simulink model "TCGreen"  (R2024b)
settings: Solver=ode45  StartTime=0.0  StopTime=1  RelTol=1e-3
undefined symbols (not defined in the file or in its folder): Cf, F, Kic, Kiv, Kpc, Kpv, Lc, Lf, Lline, mp, nq, rc, rf, Rline, Rload, Ts, Vdc, Vn, wc, wn
libraries: spsFourierLib x18, spsabctodq0Lib x14, spsThreePhaseSeriesRLCBranchLib x13, spsThreePhaseVIMeasurementLib x11, spsGroundLib x5, simulink x3, spsDCVoltageSourceLib x3, spsUniversalBridgeLib x3, spsdq0toabcLib x3, sps_lib x1
settings Model: Creator=RDP  LastModifiedBy=DAS'BEAST
settings DataIOCC: ReturnWorkspaceOutputs=off
settings RTWCC: GPUComputeCapability=3.5

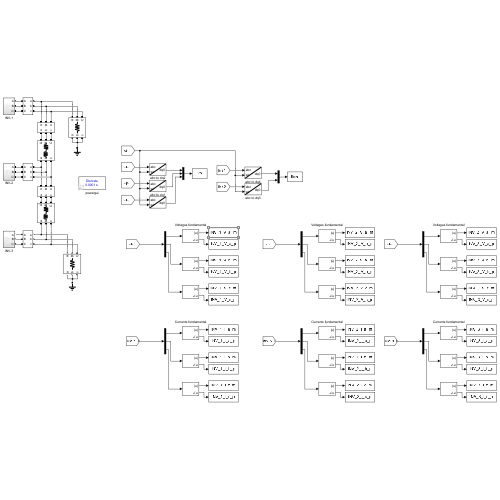
[thumbnail: Simulink's stored preview of the top-level diagram]
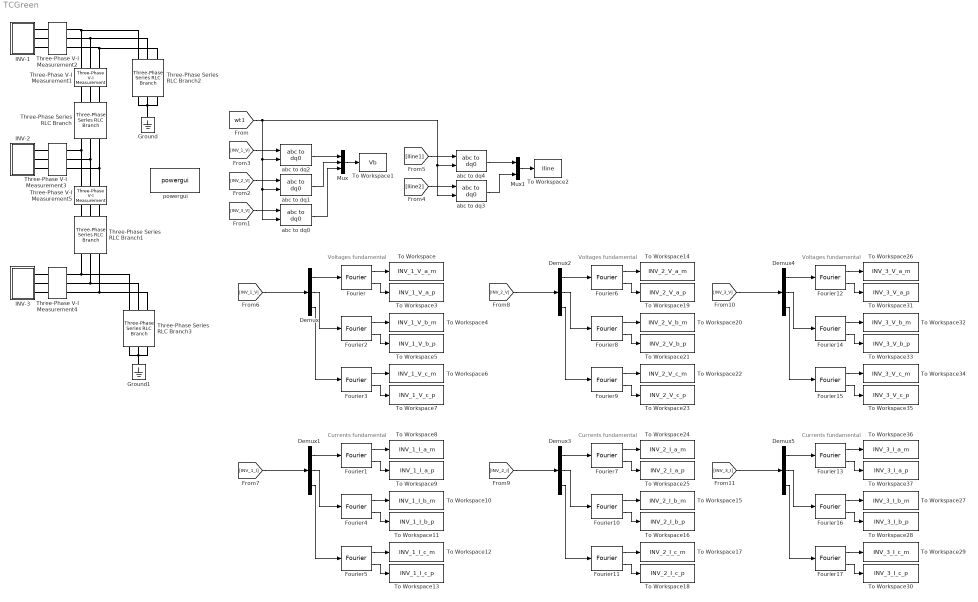
== system TCGreen ==
  note: Voltages fundamental
  note: Currents fundamental
  note: Currents fundamental
  note: Voltages fundamental
  note: Currents fundamental
  note: Voltages fundamental
  Demux{,1..5} (6 alike) : Demux  Outputs=3
  Fourier{,1..17} (18 alike) : spsFourierLib/Fourier  Freq=50  n=1  InInit=[0, 0]  Ts=0
  Ground : spsGroundLib/Ground  LConnTagsString=a
  Ground1 : spsGroundLib/Ground  LConnTagsString=a
  INV-1 : Subsystem
  INV-2 : Subsystem
  INV-3 : Subsystem
  Mux : Mux  Inputs=3
  Mux1 : Mux  Inputs=2
  Three-Phase Series RLC Branch : spsThreePhaseSeriesRLCBranchLib/Three-Phase Series RLC Branch  LConnTagsString=A|B|C  RConnTagsString=A|B|C  BranchType=RL  Resistance=Rline(1)  Inductance=Lline(1)  Capacitance=1e-6  Measurements=None
  Three-Phase Series RLC Branch1 : spsThreePhaseSeriesRLCBranchLib/Three-Phase Series RLC Branch  LConnTagsString=A|B|C  RConnTagsString=A|B|C  BranchType=RL  Resistance=Rline(2)  Inductance=Lline(2)  Capacitance=1e-6  Measurements=None
  Three-Phase Series RLC Branch2 : spsThreePhaseSeriesRLCBranchLib/Three-Phase Series RLC Branch  LConnTagsString=A|B|C  RConnTagsString=A|B|C  BranchType=R  Resistance=Rload(1)  Inductance=Lline(1)  Capacitance=1e-6  Measurements=None
  Three-Phase Series RLC Branch3 : spsThreePhaseSeriesRLCBranchLib/Three-Phase Series RLC Branch  LConnTagsString=A|B|C  RConnTagsString=A|B|C  BranchType=R  Resistance=Rload(2)  Inductance=Lline(1)  Capacitance=1e-6  Measurements=None
  Three-Phase V-I Measurement1 : spsThreePhaseVIMeasurementLib/Three-Phase V-I Measurement  VoltageMeasurement=no  SetLabelV=on  LabelV=Vb1  Vpu=off  VpuLL=off  CurrentMeasurement=yes  SetLabelI=on  LabelI=Iline1  Ipu=off  Pbase=100e6  Vbase=500e3  OutputType=Complex  PhasorSimulation=off  PSBequivalent=0
  Three-Phase V-I Measurement2 : spsThreePhaseVIMeasurementLib/Three-Phase V-I Measurement  VoltageMeasurement=phase-to-ground  SetLabelV=on  LabelV=INV_1_V  Vpu=off  VpuLL=off  CurrentMeasurement=yes  SetLabelI=on  LabelI=INV_1_I  Ipu=off  Pbase=100e6  Vbase=500e3  OutputType=Complex  PhasorSimulation=off  PSBequivalent=0
  Three-Phase V-I Measurement3 : spsThreePhaseVIMeasurementLib/Three-Phase V-I Measurement  VoltageMeasurement=phase-to-ground  SetLabelV=on  LabelV=INV_2_V  Vpu=off  VpuLL=off  CurrentMeasurement=yes  SetLabelI=on  LabelI=INV_2_I  Ipu=off  Pbase=100e6  Vbase=500e3  OutputType=Complex  PhasorSimulation=off  PSBequivalent=0
  Three-Phase V-I Measurement4 : spsThreePhaseVIMeasurementLib/Three-Phase V-I Measurement  VoltageMeasurement=phase-to-ground  SetLabelV=on  LabelV=INV_3_V  Vpu=off  VpuLL=off  CurrentMeasurement=yes  SetLabelI=on  LabelI=INV_3_I  Ipu=off  Pbase=100e6  Vbase=500e3  OutputType=Complex  PhasorSimulation=off  PSBequivalent=0
  Three-Phase V-I Measurement5 : spsThreePhaseVIMeasurementLib/Three-Phase V-I Measurement  VoltageMeasurement=no  SetLabelV=on  LabelV=Vb1  Vpu=off  VpuLL=off  CurrentMeasurement=yes  SetLabelI=on  LabelI=Iline2  Ipu=off  Pbase=100e6  Vbase=500e3  OutputType=Complex  PhasorSimulation=off  PSBequivalent=0
  To Workspace : ToWorkspace  VariableName=INV_1_V_a_m  SaveFormat=Timeseries  SampleTime=-1
  To Workspace1 : ToWorkspace  VariableName=Vb  SampleTime=-1
      settings: MaxDataPoints=1  Save2DSignal=2-D array (concatenate along first dimension)
  To Workspace10 : ToWorkspace  VariableName=INV_1_I_b_m  SaveFormat=Timeseries  SampleTime=-1
  To Workspace11 : ToWorkspace  VariableName=INV_1_I_b_p  SaveFormat=Timeseries  SampleTime=-1
  To Workspace12 : ToWorkspace  VariableName=INV_1_I_c_m  SaveFormat=Timeseries  SampleTime=-1
  To Workspace13 : ToWorkspace  VariableName=INV_1_I_c_p  SaveFormat=Timeseries  SampleTime=-1
  To Workspace14 : ToWorkspace  VariableName=INV_2_V_a_m  SaveFormat=Timeseries  SampleTime=-1
  To Workspace15 : ToWorkspace  VariableName=INV_2_I_b_m  SaveFormat=Timeseries  SampleTime=-1
  To Workspace16 : ToWorkspace  VariableName=INV_2_I_b_p  SaveFormat=Timeseries  SampleTime=-1
  To Workspace17 : ToWorkspace  VariableName=INV_2_I_c_m  SaveFormat=Timeseries  SampleTime=-1
  To Workspace18 : ToWorkspace  VariableName=INV_2_I_c_p  SaveFormat=Timeseries  SampleTime=-1
  To Workspace19 : ToWorkspace  VariableName=INV_2_V_a_p  SaveFormat=Timeseries  SampleTime=-1
  To Workspace2 : ToWorkspace  VariableName=Iline  SampleTime=-1
      settings: MaxDataPoints=1  Save2DSignal=2-D array (concatenate along first dimension)
  To Workspace20 : ToWorkspace  VariableName=INV_2_V_b_m  SaveFormat=Timeseries  SampleTime=-1
  To Workspace21 : ToWorkspace  VariableName=INV_2_V_b_p  SaveFormat=Timeseries  SampleTime=-1
  To Workspace22 : ToWorkspace  VariableName=INV_2_V_c_m  SaveFormat=Timeseries  SampleTime=-1
  To Workspace23 : ToWorkspace  VariableName=INV_2_V_c_p  SaveFormat=Timeseries  SampleTime=-1
  To Workspace24 : ToWorkspace  VariableName=INV_2_I_a_m  SaveFormat=Timeseries  SampleTime=-1
  To Workspace25 : ToWorkspace  VariableName=INV_2_I_a_p  SaveFormat=Timeseries  SampleTime=-1
  To Workspace26 : ToWorkspace  VariableName=INV_3_V_a_m  SaveFormat=Timeseries  SampleTime=-1
  To Workspace27 : ToWorkspace  VariableName=INV_3_I_b_m  SaveFormat=Timeseries  SampleTime=-1
  To Workspace28 : ToWorkspace  VariableName=INV_3_I_b_p  SaveFormat=Timeseries  SampleTime=-1
  To Workspace29 : ToWorkspace  VariableName=INV_3_I_c_m  SaveFormat=Timeseries  SampleTime=-1
  To Workspace3 : ToWorkspace  VariableName=INV_1_V_a_p  SaveFormat=Timeseries  SampleTime=-1
  To Workspace30 : ToWorkspace  VariableName=INV_3_I_c_p  SaveFormat=Timeseries  SampleTime=-1
  To Workspace31 : ToWorkspace  VariableName=INV_3_V_a_p  SaveFormat=Timeseries  SampleTime=-1
  To Workspace32 : ToWorkspace  VariableName=INV_3_V_b_m  SaveFormat=Timeseries  SampleTime=-1
  To Workspace33 : ToWorkspace  VariableName=INV_3_V_b_p  SaveFormat=Timeseries  SampleTime=-1
  To Workspace34 : ToWorkspace  VariableName=INV_3_V_c_m  SaveFormat=Timeseries  SampleTime=-1
  To Workspace35 : ToWorkspace  VariableName=INV_3_V_c_p  SaveFormat=Timeseries  SampleTime=-1
  To Workspace36 : ToWorkspace  VariableName=INV_3_I_a_m  SaveFormat=Timeseries  SampleTime=-1
  To Workspace37 : ToWorkspace  VariableName=INV_3_I_a_p  SaveFormat=Timeseries  SampleTime=-1
  To Workspace4 : ToWorkspace  VariableName=INV_1_V_b_m  SaveFormat=Timeseries  SampleTime=-1
  To Workspace5 : ToWorkspace  VariableName=INV_1_V_b_p  SaveFormat=Timeseries  SampleTime=-1
  To Workspace6 : ToWorkspace  VariableName=INV_1_V_c_m  SaveFormat=Timeseries  SampleTime=-1
  To Workspace7 : ToWorkspace  VariableName=INV_1_V_c_p  SaveFormat=Timeseries  SampleTime=-1
  To Workspace8 : ToWorkspace  VariableName=INV_1_I_a_m  SaveFormat=Timeseries  SampleTime=-1
  To Workspace9 : ToWorkspace  VariableName=INV_1_I_a_p  SaveFormat=Timeseries  SampleTime=-1
  abc to dq{0..4} (5 alike) : spsabctodq0Lib/abc to dq0  Alignment=90 degrees behind phase A axis
  powergui : sps_lib/powergui  Priority=1  SimulationMode=Discrete  SampleTime=Ts  frequency=60  Iterations=50  frequencyindice=0  Pbase=100e6  ErrMax=1e-4  UnitsV=kV  UnitsW=MW  buscounter=0  FunctionMessages=off  echomessages=off  EnableUseOfTLC=off  CurrentSourceSwitches=off  DisableSnubberDevices=off  DisableRonSwitches=off  DisableVfSwitches=off  DisplayEquations=off  AutomaticDiscreteSolvers=off  SolverType=Tustin/Backward Euler (TBE)  Interpol=off  ExternalGateDelay=off  methode=off  Ts=100  x0status=blocks  SPID=on  SwTol=0  HookPort=off  NonlinearTolerance=1e-4  nMaxIteration=100  ContinueOnMaxIteration=off  RestoreLinks=warning  ResistiveCurrentMeasurement=off  Frange=[0:2:500]  Ylog=off  Xlog=on  ShowGrid=off  save=off  variable=ZData  structure=0  ZoomFFT=off  StartTime=0.0  cycles=1  DisplayStyle=1  fundamental=60  FreqAxis=off  MaxFrequency=1000  frequencyindicesteady=1  RmsSteady=1  display=off
  wires:
  [INV_3_V] -> abc to dq0/1
  [INV_2_V] -> abc to dq1/1
  [INV_1_V] -> abc to dq2/1
  abc to dq2/1 -> Mux/1
  abc to dq1/1 -> Mux/2
  abc to dq0/1 -> Mux/3
  Mux/1 -> To Workspace1/1
  Mux1/1 -> To Workspace2/1
  abc to dq3/1 -> Mux1/2
  abc to dq4/1 -> Mux1/1
  [Iline1] -> abc to dq4/1
  [Iline2] -> abc to dq3/1
  [wt1] -> abc to dq3/2, abc to dq4/2, abc to dq2/2, abc to dq0/2, abc to dq1/2
  [INV_1_V] -> Demux/1
  Demux/2 -> Fourier2/1
  Demux/3 -> Fourier3/1
  Demux/1 -> Fourier/1
  Fourier/1 -> To Workspace/1
  Fourier2/1 -> To Workspace4/1
  Fourier3/1 -> To Workspace6/1
  Fourier3/2 -> To Workspace7/1
  Fourier2/2 -> To Workspace5/1
  Fourier/2 -> To Workspace3/1
  Demux1/1 -> Fourier1/1
  Demux1/2 -> Fourier4/1
  Fourier4/1 -> To Workspace10/1
  Fourier5/2 -> To Workspace13/1
  Fourier1/1 -> To Workspace8/1
  Fourier5/1 -> To Workspace12/1
  Demux1/3 -> Fourier5/1
  Fourier4/2 -> To Workspace11/1
  [INV_1_I] -> Demux1/1
  Fourier1/2 -> To Workspace9/1
  Demux2/1 -> Fourier6/1
  Demux2/2 -> Fourier8/1
  Fourier8/2 -> To Workspace21/1
  Fourier8/1 -> To Workspace20/1
  Demux3/3 -> Fourier11/1
  Fourier10/2 -> To Workspace16/1
  Fourier7/2 -> To Workspace25/1
  Fourier11/1 -> To Workspace17/1
  [INV_2_I] -> Demux3/1
  Demux3/2 -> Fourier10/1
  Fourier11/2 -> To Workspace18/1
  Fourier9/2 -> To Workspace23/1
  Fourier6/1 -> To Workspace14/1
  Demux3/1 -> Fourier7/1
  Fourier9/1 -> To Workspace22/1
  Demux2/3 -> Fourier9/1
  Fourier10/1 -> To Workspace15/1
  Fourier6/2 -> To Workspace19/1
  [INV_2_V] -> Demux2/1
  Fourier7/1 -> To Workspace24/1
  Demux4/1 -> Fourier12/1
  Demux4/2 -> Fourier14/1
  Fourier14/2 -> To Workspace33/1
  Fourier14/1 -> To Workspace32/1
  Demux5/3 -> Fourier17/1
  Fourier16/2 -> To Workspace28/1
  Fourier13/2 -> To Workspace37/1
  Fourier17/1 -> To Workspace29/1
  [INV_3_I] -> Demux5/1
  Demux5/2 -> Fourier16/1
  Fourier17/2 -> To Workspace30/1
  Fourier15/2 -> To Workspace35/1
  Fourier12/1 -> To Workspace26/1
  Demux5/1 -> Fourier13/1
  Fourier15/1 -> To Workspace34/1
  Demux4/3 -> Fourier15/1
  Fourier16/1 -> To Workspace27/1
  Fourier12/2 -> To Workspace31/1
  [INV_3_V] -> Demux4/1
  Fourier13/1 -> To Workspace36/1
  connections:
  Three-Phase Series RLC Branch2/LConn1 -- Three-Phase V-I Measurement2/RConn1 -- Three-Phase V-I Measurement1/LConn1
  Three-Phase V-I Measurement2/RConn2 -- Three-Phase V-I Measurement1/LConn2 -- Three-Phase Series RLC Branch2/LConn2
  Three-Phase Series RLC Branch2/LConn3 -- Three-Phase V-I Measurement1/LConn3 -- Three-Phase V-I Measurement2/RConn3
  Three-Phase V-I Measurement3/RConn1 -- Three-Phase V-I Measurement5/LConn1 -- Three-Phase Series RLC Branch/RConn1
  Three-Phase V-I Measurement3/RConn2 -- Three-Phase V-I Measurement5/LConn2 -- Three-Phase Series RLC Branch/RConn2
  Three-Phase V-I Measurement3/RConn3 -- Three-Phase V-I Measurement5/LConn3 -- Three-Phase Series RLC Branch/RConn3
  Three-Phase Series RLC Branch2/RConn1 -- Ground/LConn1 -- Three-Phase Series RLC Branch2/RConn2 -- Three-Phase Series RLC Branch2/RConn3
  Three-Phase Series RLC Branch1/RConn1 -- Three-Phase Series RLC Branch3/LConn1 -- Three-Phase V-I Measurement4/RConn1
  Three-Phase Series RLC Branch1/RConn2 -- Three-Phase V-I Measurement4/RConn2 -- Three-Phase Series RLC Branch3/LConn2
  Three-Phase Series RLC Branch1/RConn3 -- Three-Phase Series RLC Branch3/LConn3 -- Three-Phase V-I Measurement4/RConn3
  Three-Phase Series RLC Branch3/RConn1 -- Ground1/LConn1 -- Three-Phase Series RLC Branch3/RConn2 -- Three-Phase Series RLC Branch3/RConn3
  INV-1/RConn1 -- Three-Phase V-I Measurement2/LConn1
  INV-1/RConn2 -- Three-Phase V-I Measurement2/LConn2
  INV-1/RConn3 -- Three-Phase V-I Measurement2/LConn3
  Three-Phase V-I Measurement3/LConn1 -- INV-2/RConn1
  Three-Phase V-I Measurement3/LConn2 -- INV-2/RConn2
  Three-Phase V-I Measurement3/LConn3 -- INV-2/RConn3
  Three-Phase V-I Measurement4/LConn1 -- INV-3/RConn1
  Three-Phase V-I Measurement4/LConn2 -- INV-3/RConn2
  Three-Phase V-I Measurement4/LConn3 -- INV-3/RConn3
  Three-Phase V-I Measurement1/RConn1 -- Three-Phase Series RLC Branch/LConn1
  Three-Phase Series RLC Branch/LConn2 -- Three-Phase V-I Measurement1/RConn2
  Three-Phase V-I Measurement1/RConn3 -- Three-Phase Series RLC Branch/LConn3
  Three-Phase V-I Measurement5/RConn1 -- Three-Phase Series RLC Branch1/LConn1
  Three-Phase V-I Measurement5/RConn2 -- Three-Phase Series RLC Branch1/LConn2
  Three-Phase V-I Measurement5/RConn3 -- Three-Phase Series RLC Branch1/LConn3

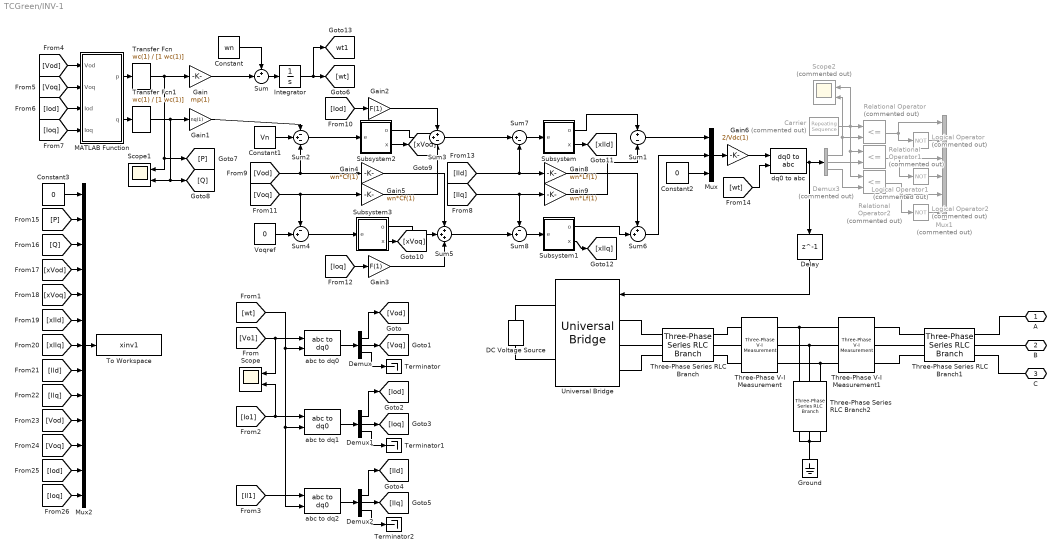
== system TCGreen/INV-1 ==
  Carrier : simulink/Sources/Repeating Sequence  Commented=on  rep_seq_t=[0 0.5 1]/10000  rep_seq_y=[-1 1 -1]
  Constant : Constant  Value=wn
  Constant1 : Constant  Value=Vn
  Constant2 : Constant  Value=0
  Constant3 : Constant  Value=0
  DC Voltage Source : spsDCVoltageSourceLib/DC Voltage Source  Amplitude=Vdc(1)  Measurements=None
  Delay : Delay  DelayLength=1
  Demux : Demux  Outputs=3
  Demux1 : Demux  Outputs=3
  Demux2 : Demux  Outputs=3
  Demux3 : Demux  Commented=on  Outputs=3
  Gain : Gain  Gain=mp(1)
  Gain1 : Gain  Gain=nq(1)
  Gain2 : Gain  Gain=F(1)
  Gain3 : Gain  Gain=F(1)
  Gain4 : Gain  Gain=wn*Cf(1)
  Gain5 : Gain  Gain=wn*Cf(1)
  Gain6 : Gain  Gain=2/Vdc(1)
  Gain8 : Gain  Gain=wn*Lf(1)
  Gain9 : Gain  Gain=wn*Lf(1)
  Ground : spsGroundLib/Ground  LConnTagsString=a
  Integrator : Integrator  WrappedStateUpperValue=2*pi  WrappedStateLowerValue=0
  Logical Operator : Logic  Commented=on  Operator=NOT  IconShape=distinctive  AllPortsSameDT=off  OutDataTypeStr=boolean
  Logical Operator1 : Logic  Commented=on  Operator=NOT  IconShape=distinctive  AllPortsSameDT=off  OutDataTypeStr=boolean
  Logical Operator2 : Logic  Commented=on  Operator=NOT  IconShape=distinctive  AllPortsSameDT=off  OutDataTypeStr=boolean
  MATLAB Function : MATLAB Function  TreatAsAtomicUnit=on
  Mux : Mux  Inputs=3
  Mux1 : Mux  Commented=on  Inputs=6
  Mux2 : Mux  Inputs=13
  Relational Operator : RelationalOperator  Commented=on  Operator=<=  OutDataTypeStr=boolean  RndMeth=Simplest  InputSameDT=off
  Relational Operator1 : RelationalOperator  Commented=on  Operator=<=  OutDataTypeStr=boolean  RndMeth=Simplest  InputSameDT=off
  Relational Operator2 : RelationalOperator  Commented=on  Operator=<=  OutDataTypeStr=boolean  RndMeth=Simplest  InputSameDT=off
  Scope : Scope  NumInputPorts=2
  Scope1 : Scope  NumInputPorts=2
  Scope2 : Scope  Commented=on  NumInputPorts=2
  Subsystem : Subsystem
  Subsystem1 : Subsystem
  Subsystem2 : Subsystem
  Subsystem3 : Subsystem
  Sum : Sum  Inputs=+-|
  Sum1 : Sum  Inputs=+-
  Sum2 : Sum  Inputs=-+-
  Sum3 : Sum  Inputs=++-
  Sum4 : Sum  Inputs=-+|
  Sum5 : Sum  Inputs=+++
  Sum6 : Sum  Inputs=++|
  Sum7 : Sum  Inputs=|+-
  Sum8 : Sum  Inputs=-+|
  Terminator : Terminator
  Terminator1 : Terminator
  Terminator2 : Terminator
  Three-Phase Series RLC Branch : spsThreePhaseSeriesRLCBranchLib/Three-Phase Series RLC Branch  LConnTagsString=A|B|C  RConnTagsString=A|B|C  BranchType=RL  Resistance=rf(1)  Inductance=Lf(1)  Capacitance=1e-6  Measurements=None
  Three-Phase Series RLC Branch1 : spsThreePhaseSeriesRLCBranchLib/Three-Phase Series RLC Branch  LConnTagsString=A|B|C  RConnTagsString=A|B|C  BranchType=RL  Resistance=rc(1)  Inductance=Lc(1)  Capacitance=1e-6  Measurements=None
  Three-Phase Series RLC Branch2 : spsThreePhaseSeriesRLCBranchLib/Three-Phase Series RLC Branch  LConnTagsString=A|B|C  RConnTagsString=A|B|C  BranchType=C  Resistance=rf(1)  Inductance=Lf(1)  Capacitance=Cf(1)  Measurements=None
  Three-Phase V-I Measurement : spsThreePhaseVIMeasurementLib/Three-Phase V-I Measurement  VoltageMeasurement=no  SetLabelV=off  LabelV=Vabc  Vpu=off  VpuLL=off  CurrentMeasurement=yes  SetLabelI=on  LabelI=Il1  Ipu=off  Pbase=100e6  Vbase=500e3  OutputType=Complex  PhasorSimulation=off  PSBequivalent=0
  Three-Phase V-I Measurement1 : spsThreePhaseVIMeasurementLib/Three-Phase V-I Measurement  VoltageMeasurement=phase-to-ground  SetLabelV=on  LabelV=Vo1  Vpu=off  VpuLL=off  CurrentMeasurement=yes  SetLabelI=on  LabelI=Io1  Ipu=off  Pbase=100e6  Vbase=500e3  OutputType=Complex  PhasorSimulation=off  PSBequivalent=0
  To Workspace : ToWorkspace  VariableName=xinv1  SampleTime=-1
      settings: MaxDataPoints=1  Save2DSignal=2-D array (concatenate along first dimension)
  Transfer Fcn : TransferFcn  Numerator=wc(1)  Denominator=[1 wc(1)]
  Transfer Fcn1 : TransferFcn  Numerator=wc(1)  Denominator=[1 wc(1)]
  Universal Bridge : spsUniversalBridgeLib/Universal Bridge  Arms=3  SnubberResistance=1e5  SnubberCapacitance=inf  Device=Average-model based VSC  Ron=1e-3  Lon=0  ForwardVoltages="[  0  0  ]"  ForwardVoltage=0  GTOparameters=[ 10e-6 , 20e-6 ]  IGBTparameters=[ 1e-6 , 2e-6 ]  Measurements=None  Measurements_2=None  converterType=Rectifier
  Voqref : Constant  Value=0
  abc to dq0 : spsabctodq0Lib/abc to dq0  Alignment=90 degrees behind phase A axis
  abc to dq1 : spsabctodq0Lib/abc to dq0  Alignment=90 degrees behind phase A axis
  abc to dq2 : spsabctodq0Lib/abc to dq0  Alignment=90 degrees behind phase A axis
  dq0 to abc : spsdq0toabcLib/dq0 to abc  Alignment=90 degrees behind phase A axis
  A : PMIOPort  Side=Right
  B : PMIOPort  Port=2  Side=Right
  C : PMIOPort  Port=3  Side=Right
  tag scope: wt1=global
  wires:
  [Vo1] -> Scope/1, abc to dq0/1
  abc to dq0/1 -> Demux/1
  Demux/1 -> [Vod]
  Demux/2 -> [Voq]
  Demux/3 -> Terminator/1
  Demux1/3 -> Terminator1/1
  Demux1/2 -> [Ioq]
  Demux1/1 -> [Iod]
  abc to dq1/1 -> Demux1/1
  [Io1] -> Scope/2, abc to dq1/1
  [Il1] -> abc to dq2/1
  Demux2/1 -> [Ild]
  abc to dq2/1 -> Demux2/1
  Demux2/2 -> [Ilq]
  Demux2/3 -> Terminator2/1
  [wt] -> abc to dq0/2, abc to dq1/2, abc to dq2/2
  [Voq] -> MATLAB Function/2(Voq)
  [Vod] -> MATLAB Function/1(Vod)
  [Iod] -> MATLAB Function/3(Iod)
  [Ioq] -> MATLAB Function/4(Ioq)
  MATLAB Function/1(p) -> Transfer Fcn/1
  MATLAB Function/2(q) -> Transfer Fcn1/1
  Transfer Fcn/1 -> Scope1/1, [P], Gain/1
  Constant/1 -> Sum/1
  Transfer Fcn1/1 -> [Q], Scope1/2, Gain1/1
  Sum/1 -> Integrator/1
  Integrator/1 -> [wt], [wt1]
  [Vod] -> Sum2/3, Gain4/1
  Sum2/1 -> Subsystem2/1(e)
  Subsystem2/1(o) -> Sum3/2
  [Iod] -> Gain2/1
  Gain2/1 -> Sum3/1
  Voqref/1 -> Sum4/2
  [Voq] -> Gain5/1, Sum4/1
  Sum4/1 -> Subsystem3/1(e)
  Subsystem3/1(o) -> Sum5/2
  [Ioq] -> Gain3/1
  Gain3/1 -> Sum5/3
  Gain4/1 -> Sum5/1
  Gain5/1 -> Sum3/3
  Constant1/1 -> Sum2/2
  Gain8/1 -> Sum6/1
  Subsystem1/1(o) -> Sum6/2
  [Ilq] -> Sum8/1, Gain9/1
  [Ild] -> Sum7/2, Gain8/1
  Subsystem/1(o) -> Sum1/1
  Gain9/1 -> Sum1/2
  Sum3/1 -> Sum7/1
  Sum5/1 -> Sum8/2
  Sum7/1 -> Subsystem/1(e)
  Sum8/1 -> Subsystem1/1(e)
  Sum1/1 -> Mux/1
  Sum6/1 -> Mux/2
  Constant2/1 -> Mux/3
  Mux/1 -> Gain6/1
  Gain6/1 -> dq0 to abc/1
  [wt] -> dq0 to abc/2
  dq0 to abc/1 -> Demux3/1, Delay/1
  Demux3/1 -> Scope2/2, Relational Operator/2
  Demux3/2 -> Relational Operator1/2
  Demux3/3 -> Relational Operator2/2
  Carrier/1 -> Scope2/1, Relational Operator2/1, Relational Operator1/1, Relational Operator/1
  Relational Operator/1 -> Logical Operator/1, Mux1/1
  Relational Operator1/1 -> Logical Operator1/1, Mux1/3
  Relational Operator2/1 -> Logical Operator2/1, Mux1/5
  Logical Operator/1 -> Mux1/2
  Logical Operator1/1 -> Mux1/4
  Logical Operator2/1 -> Mux1/6
  Gain/1 -> Sum/2
  Gain1/1 -> Sum2/1
  Constant3/1 -> Mux2/1
  [P] -> Mux2/2
  [Q] -> Mux2/3
  [xVod] -> Mux2/4
  [xVoq] -> Mux2/5
  [xIld] -> Mux2/6
  [xIlq] -> Mux2/7
  [Ild] -> Mux2/8
  [Ilq] -> Mux2/9
  [Vod] -> Mux2/10
  [Voq] -> Mux2/11
  [Iod] -> Mux2/12
  [Ioq] -> Mux2/13
  Mux2/1 -> To Workspace/1
  Delay/1 -> Universal Bridge/1
  Subsystem/2(x) -> [xIld]
  Subsystem1/2(x) -> [xIlq]
  Subsystem2/2(x) -> [xVod]
  Subsystem3/2(x) -> [xVoq]
  connections:
  Three-Phase Series RLC Branch/LConn3 -- Universal Bridge/LConn3
  Three-Phase V-I Measurement/LConn3 -- Three-Phase Series RLC Branch/RConn3
  Three-Phase Series RLC Branch/RConn2 -- Three-Phase V-I Measurement/LConn2
  Three-Phase Series RLC Branch1/RConn3 -- C/RConn1
  Three-Phase Series RLC Branch/LConn2 -- Universal Bridge/LConn2
  Three-Phase V-I Measurement1/LConn2 -- Three-Phase V-I Measurement/RConn2 -- Three-Phase Series RLC Branch2/LConn2
  DC Voltage Source/RConn1 -- Universal Bridge/RConn1
  Three-Phase Series RLC Branch1/RConn2 -- B/RConn1
  Three-Phase V-I Measurement1/LConn1 -- Three-Phase V-I Measurement/RConn1 -- Three-Phase Series RLC Branch2/LConn1
  Three-Phase Series RLC Branch1/LConn1 -- Three-Phase V-I Measurement1/RConn1
  DC Voltage Source/LConn1 -- Universal Bridge/RConn2
  Three-Phase Series RLC Branch1/LConn2 -- Three-Phase V-I Measurement1/RConn2
  Three-Phase Series RLC Branch2/RConn1 -- Ground/LConn1 -- Three-Phase Series RLC Branch2/RConn2 -- Three-Phase Series RLC Branch2/RConn3
  Three-Phase V-I Measurement1/LConn3 -- Three-Phase V-I Measurement/RConn3 -- Three-Phase Series RLC Branch2/LConn3
  Universal Bridge/LConn1 -- Three-Phase Series RLC Branch/LConn1
  Three-Phase V-I Measurement/LConn1 -- Three-Phase Series RLC Branch/RConn1
  Three-Phase V-I Measurement1/RConn3 -- Three-Phase Series RLC Branch1/LConn3
  Three-Phase Series RLC Branch1/RConn1 -- A/RConn1

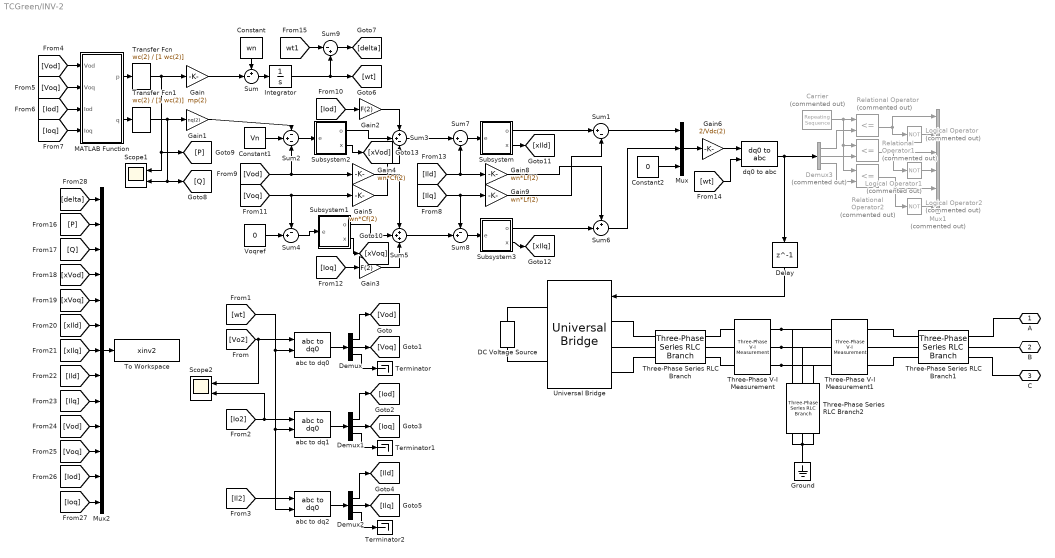
== system TCGreen/INV-2 ==
  Carrier : simulink/Sources/Repeating Sequence  Commented=on  rep_seq_t=[0 0.5 1]/10000  rep_seq_y=[-1 1 -1]
  Constant : Constant  Value=wn
  Constant1 : Constant  Value=Vn
  Constant2 : Constant  Value=0
  DC Voltage Source : spsDCVoltageSourceLib/DC Voltage Source  Amplitude=Vdc(2)  Measurements=None
  Delay : Delay  DelayLength=1
  Demux : Demux  Outputs=3
  Demux1 : Demux  Outputs=3
  Demux2 : Demux  Outputs=3
  Demux3 : Demux  Commented=on  Outputs=3
  Gain : Gain  Gain=mp(2)
  Gain1 : Gain  Gain=nq(2)
  Gain2 : Gain  Gain=F(2)
  Gain3 : Gain  Gain=F(2)
  Gain4 : Gain  Gain=wn*Cf(2)
  Gain5 : Gain  Gain=wn*Cf(2)
  Gain6 : Gain  Gain=2/Vdc(2)
  Gain8 : Gain  Gain=wn*Lf(2)
  Gain9 : Gain  Gain=wn*Lf(2)
  Ground : spsGroundLib/Ground  LConnTagsString=a
  Integrator : Integrator  WrappedStateUpperValue=2*pi  WrappedStateLowerValue=0
  Logical Operator : Logic  Commented=on  Operator=NOT  IconShape=distinctive  AllPortsSameDT=off  OutDataTypeStr=boolean
  Logical Operator1 : Logic  Commented=on  Operator=NOT  IconShape=distinctive  AllPortsSameDT=off  OutDataTypeStr=boolean
  Logical Operator2 : Logic  Commented=on  Operator=NOT  IconShape=distinctive  AllPortsSameDT=off  OutDataTypeStr=boolean
  MATLAB Function : MATLAB Function  TreatAsAtomicUnit=on
  Mux : Mux  Inputs=3
  Mux1 : Mux  Commented=on  Inputs=6
  Mux2 : Mux  Inputs=13
  Relational Operator : RelationalOperator  Commented=on  Operator=<=  OutDataTypeStr=boolean  RndMeth=Simplest  InputSameDT=off
  Relational Operator1 : RelationalOperator  Commented=on  Operator=<=  OutDataTypeStr=boolean  RndMeth=Simplest  InputSameDT=off
  Relational Operator2 : RelationalOperator  Commented=on  Operator=<=  OutDataTypeStr=boolean  RndMeth=Simplest  InputSameDT=off
  Scope1 : Scope  NumInputPorts=2
  Scope2 : Scope  NumInputPorts=2
  Subsystem : Subsystem
  Subsystem1 : Subsystem
  Subsystem2 : Subsystem
  Subsystem3 : Subsystem
  Sum : Sum  Inputs=+-|
  Sum1 : Sum  Inputs=|+-
  Sum2 : Sum  Inputs=-+-
  Sum3 : Sum  Inputs=++-
  Sum4 : Sum  Inputs=-+|
  Sum5 : Sum  Inputs=+++
  Sum6 : Sum  Inputs=++|
  Sum7 : Sum  Inputs=|+-
  Sum8 : Sum  Inputs=-+|
  Sum9 : Sum  Inputs=|-+
  Terminator : Terminator
  Terminator1 : Terminator
  Terminator2 : Terminator
  Three-Phase Series RLC Branch : spsThreePhaseSeriesRLCBranchLib/Three-Phase Series RLC Branch  LConnTagsString=A|B|C  RConnTagsString=A|B|C  BranchType=RL  Resistance=rf(2)  Inductance=Lf(2)  Capacitance=1e-6  Measurements=None
  Three-Phase Series RLC Branch1 : spsThreePhaseSeriesRLCBranchLib/Three-Phase Series RLC Branch  LConnTagsString=A|B|C  RConnTagsString=A|B|C  BranchType=RL  Resistance=rc(2)  Inductance=Lc(2)  Capacitance=1e-6  Measurements=None
  Three-Phase Series RLC Branch2 : spsThreePhaseSeriesRLCBranchLib/Three-Phase Series RLC Branch  LConnTagsString=A|B|C  RConnTagsString=A|B|C  BranchType=C  Resistance=rf(1)  Inductance=Lf(1)  Capacitance=Cf(2)  Measurements=None
  Three-Phase V-I Measurement : spsThreePhaseVIMeasurementLib/Three-Phase V-I Measurement  VoltageMeasurement=no  SetLabelV=off  LabelV=Vabc  Vpu=off  VpuLL=off  CurrentMeasurement=yes  SetLabelI=on  LabelI=Il2  Ipu=off  Pbase=100e6  Vbase=500e3  OutputType=Complex  PhasorSimulation=off  PSBequivalent=0
  Three-Phase V-I Measurement1 : spsThreePhaseVIMeasurementLib/Three-Phase V-I Measurement  VoltageMeasurement=phase-to-ground  SetLabelV=on  LabelV=Vo2  Vpu=off  VpuLL=off  CurrentMeasurement=yes  SetLabelI=on  LabelI=Io2  Ipu=off  Pbase=100e6  Vbase=500e3  OutputType=Complex  PhasorSimulation=off  PSBequivalent=0
  To Workspace : ToWorkspace  VariableName=xinv2  SampleTime=-1
      settings: MaxDataPoints=1  Save2DSignal=2-D array (concatenate along first dimension)
  Transfer Fcn : TransferFcn  Numerator=wc(2)  Denominator=[1 wc(2)]
  Transfer Fcn1 : TransferFcn  Numerator=wc(2)  Denominator=[1 wc(2)]
  Universal Bridge : spsUniversalBridgeLib/Universal Bridge  Arms=3  SnubberResistance=1e5  SnubberCapacitance=inf  Device=Average-model based VSC  Ron=1e-3  Lon=0  ForwardVoltages="[  0  0  ]"  ForwardVoltage=0  GTOparameters=[ 10e-6 , 20e-6 ]  IGBTparameters=[ 1e-6 , 2e-6 ]  Measurements=None  Measurements_2=None  converterType=Rectifier
  Voqref : Constant  Value=0
  abc to dq0 : spsabctodq0Lib/abc to dq0  Alignment=90 degrees behind phase A axis
  abc to dq1 : spsabctodq0Lib/abc to dq0  Alignment=90 degrees behind phase A axis
  abc to dq2 : spsabctodq0Lib/abc to dq0  Alignment=90 degrees behind phase A axis
  dq0 to abc : spsdq0toabcLib/dq0 to abc  Alignment=90 degrees behind phase A axis
  A : PMIOPort  Side=Right
  B : PMIOPort  Port=2  Side=Right
  C : PMIOPort  Port=3  Side=Right
  wires:
  Logical Operator2/1 -> Mux1/6
  Logical Operator1/1 -> Mux1/4
  Logical Operator/1 -> Mux1/2
  Relational Operator2/1 -> Mux1/5, Logical Operator2/1
  Relational Operator1/1 -> Mux1/3, Logical Operator1/1
  Relational Operator/1 -> Mux1/1, Logical Operator/1
  Carrier/1 -> Relational Operator/1, Relational Operator1/1, Relational Operator2/1
  Demux3/3 -> Relational Operator2/2
  Demux3/2 -> Relational Operator1/2
  Demux3/1 -> Relational Operator/2
  dq0 to abc/1 -> Delay/1, Demux3/1
  [wt] -> dq0 to abc/2
  Mux/1 -> Gain6/1
  Constant2/1 -> Mux/3
  Sum6/1 -> Mux/2
  Sum1/1 -> Mux/1
  Sum8/1 -> Subsystem3/1(e)
  Sum7/1 -> Subsystem/1(e)
  Sum5/1 -> Sum8/2
  Sum3/1 -> Sum7/1
  Gain9/1 -> Sum1/2
  Subsystem/1(o) -> Sum1/1
  [Ild] -> Gain8/1, Sum7/2
  [Ilq] -> Gain9/1, Sum8/1
  Subsystem3/1(o) -> Sum6/2
  Gain8/1 -> Sum6/1
  Constant1/1 -> Sum2/2
  Gain5/1 -> Sum3/3
  Gain4/1 -> Sum5/1
  Gain3/1 -> Sum5/3
  [Ioq] -> Gain3/1
  Subsystem1/1(o) -> Sum5/2
  Sum4/1 -> Subsystem1/1(e)
  [Voq] -> Sum4/1, Gain5/1
  Voqref/1 -> Sum4/2
  Gain2/1 -> Sum3/1
  [Iod] -> Gain2/1
  Subsystem2/1(o) -> Sum3/2
  Sum2/1 -> Subsystem2/1(e)
  [Vod] -> Gain4/1, Sum2/3
  Integrator/1 -> Sum9/2, [wt]
  Sum/1 -> Integrator/1
  Constant/1 -> Sum/1
  MATLAB Function/2(q) -> Transfer Fcn1/1
  MATLAB Function/1(p) -> Transfer Fcn/1
  [Ioq] -> MATLAB Function/4(Ioq)
  [Iod] -> MATLAB Function/3(Iod)
  [Vod] -> MATLAB Function/1(Vod)
  [Voq] -> MATLAB Function/2(Voq)
  [wt] -> abc to dq2/2, abc to dq1/2, abc to dq0/2
  Demux2/3 -> Terminator2/1
  Demux2/2 -> [Ilq]
  abc to dq2/1 -> Demux2/1
  Demux2/1 -> [Ild]
  [Il2] -> abc to dq2/1
  [Io2] -> Scope2/2, abc to dq1/1
  abc to dq1/1 -> Demux1/1
  Demux1/1 -> [Iod]
  Demux1/2 -> [Ioq]
  Demux1/3 -> Terminator1/1
  Demux/3 -> Terminator/1
  Demux/2 -> [Voq]
  Demux/1 -> [Vod]
  abc to dq0/1 -> Demux/1
  [Vo2] -> Scope2/1, abc to dq0/1
  Gain/1 -> Sum/2
  Transfer Fcn1/1 -> [Q], Scope1/2, Gain1/1
  Transfer Fcn/1 -> [P], Scope1/1, Gain/1
  Gain1/1 -> Sum2/1
  [wt1] -> Sum9/1
  Sum9/1 -> [delta]
  [xVoq] -> Mux2/5
  [xIlq] -> Mux2/7
  [Ioq] -> Mux2/13
  [Iod] -> Mux2/12
  [Voq] -> Mux2/11
  [Ild] -> Mux2/8
  [xIld] -> Mux2/6
  [Q] -> Mux2/3
  [P] -> Mux2/2
  [xVod] -> Mux2/4
  [Ilq] -> Mux2/9
  [delta] -> Mux2/1
  Mux2/1 -> To Workspace/1
  [Vod] -> Mux2/10
  Gain6/1 -> dq0 to abc/1
  Delay/1 -> Universal Bridge/1
  Subsystem2/2(x) -> [xVod]
  Subsystem1/2(x) -> [xVoq]
  Subsystem/2(x) -> [xIld]
  Subsystem3/2(x) -> [xIlq]
  connections:
  Three-Phase Series RLC Branch1/RConn1 -- A/RConn1
  Three-Phase V-I Measurement1/RConn3 -- Three-Phase Series RLC Branch1/LConn3
  Three-Phase V-I Measurement/LConn1 -- Three-Phase Series RLC Branch/RConn1
  Universal Bridge/LConn1 -- Three-Phase Series RLC Branch/LConn1
  Three-Phase V-I Measurement/RConn3 -- Three-Phase V-I Measurement1/LConn3 -- Three-Phase Series RLC Branch2/LConn3
  Ground/LConn1 -- Three-Phase Series RLC Branch2/RConn3 -- Three-Phase Series RLC Branch2/RConn1 -- Three-Phase Series RLC Branch2/RConn2
  Three-Phase Series RLC Branch1/LConn2 -- Three-Phase V-I Measurement1/RConn2
  DC Voltage Source/LConn1 -- Universal Bridge/RConn2
  Three-Phase Series RLC Branch1/LConn1 -- Three-Phase V-I Measurement1/RConn1
  Three-Phase V-I Measurement/RConn1 -- Three-Phase V-I Measurement1/LConn1 -- Three-Phase Series RLC Branch2/LConn1
  Three-Phase Series RLC Branch1/RConn2 -- B/RConn1
  DC Voltage Source/RConn1 -- Universal Bridge/RConn1
  Three-Phase V-I Measurement/RConn2 -- Three-Phase V-I Measurement1/LConn2 -- Three-Phase Series RLC Branch2/LConn2
  Three-Phase Series RLC Branch/LConn2 -- Universal Bridge/LConn2
  Three-Phase Series RLC Branch1/RConn3 -- C/RConn1
  Three-Phase Series RLC Branch/RConn2 -- Three-Phase V-I Measurement/LConn2
  Three-Phase V-I Measurement/LConn3 -- Three-Phase Series RLC Branch/RConn3
  Three-Phase Series RLC Branch/LConn3 -- Universal Bridge/LConn3

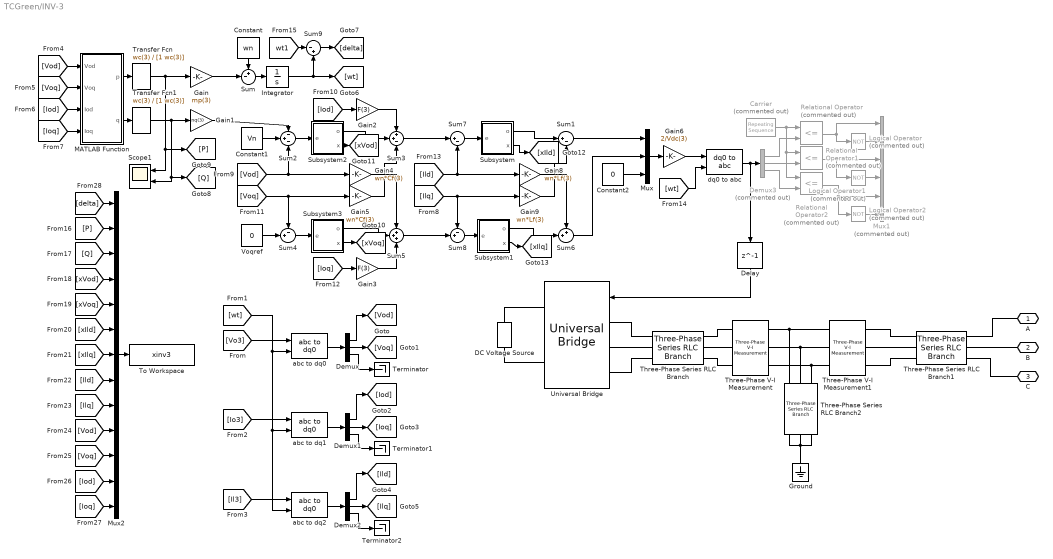
== system TCGreen/INV-3 ==
  Carrier : simulink/Sources/Repeating Sequence  Commented=on  rep_seq_t=[0 0.5 1]/10000  rep_seq_y=[-1 1 -1]
  Constant : Constant  Value=wn
  Constant1 : Constant  Value=Vn
  Constant2 : Constant  Value=0
  DC Voltage Source : spsDCVoltageSourceLib/DC Voltage Source  Amplitude=Vdc(3)  Measurements=None
  Delay : Delay  DelayLength=1
  Demux : Demux  Outputs=3
  Demux1 : Demux  Outputs=3
  Demux2 : Demux  Outputs=3
  Demux3 : Demux  Commented=on  Outputs=3
  Gain : Gain  Gain=mp(3)
  Gain1 : Gain  Gain=nq(3)
  Gain2 : Gain  Gain=F(3)
  Gain3 : Gain  Gain=F(3)
  Gain4 : Gain  Gain=wn*Cf(3)
  Gain5 : Gain  Gain=wn*Cf(3)
  Gain6 : Gain  Gain=2/Vdc(3)
  Gain8 : Gain  Gain=wn*Lf(3)
  Gain9 : Gain  Gain=wn*Lf(3)
  Ground : spsGroundLib/Ground  LConnTagsString=a
  Integrator : Integrator  WrappedStateUpperValue=2*pi  WrappedStateLowerValue=0
  Logical Operator : Logic  Commented=on  Operator=NOT  IconShape=distinctive  AllPortsSameDT=off  OutDataTypeStr=boolean
  Logical Operator1 : Logic  Commented=on  Operator=NOT  IconShape=distinctive  AllPortsSameDT=off  OutDataTypeStr=boolean
  Logical Operator2 : Logic  Commented=on  Operator=NOT  IconShape=distinctive  AllPortsSameDT=off  OutDataTypeStr=boolean
  MATLAB Function : MATLAB Function  TreatAsAtomicUnit=on
  Mux : Mux  Inputs=3
  Mux1 : Mux  Commented=on  Inputs=6
  Mux2 : Mux  Inputs=13
  Relational Operator : RelationalOperator  Commented=on  Operator=<=  OutDataTypeStr=boolean  RndMeth=Simplest  InputSameDT=off
  Relational Operator1 : RelationalOperator  Commented=on  Operator=<=  OutDataTypeStr=boolean  RndMeth=Simplest  InputSameDT=off
  Relational Operator2 : RelationalOperator  Commented=on  Operator=<=  OutDataTypeStr=boolean  RndMeth=Simplest  InputSameDT=off
  Scope1 : Scope  NumInputPorts=2
  Subsystem : Subsystem
  Subsystem1 : Subsystem
  Subsystem2 : Subsystem
  Subsystem3 : Subsystem
  Sum : Sum  Inputs=+-|
  Sum1 : Sum  Inputs=|+-
  Sum2 : Sum  Inputs=-+-
  Sum3 : Sum  Inputs=++-
  Sum4 : Sum  Inputs=-+|
  Sum5 : Sum  Inputs=+++
  Sum6 : Sum  Inputs=++|
  Sum7 : Sum  Inputs=|+-
  Sum8 : Sum  Inputs=-+|
  Sum9 : Sum  Inputs=|-+
  Terminator : Terminator
  Terminator1 : Terminator
  Terminator2 : Terminator
  Three-Phase Series RLC Branch : spsThreePhaseSeriesRLCBranchLib/Three-Phase Series RLC Branch  LConnTagsString=A|B|C  RConnTagsString=A|B|C  BranchType=RL  Resistance=rf(3)  Inductance=Lf(3)  Capacitance=1e-6  Measurements=None
  Three-Phase Series RLC Branch1 : spsThreePhaseSeriesRLCBranchLib/Three-Phase Series RLC Branch  LConnTagsString=A|B|C  RConnTagsString=A|B|C  BranchType=RL  Resistance=rc(3)  Inductance=Lc(3)  Capacitance=1e-6  Measurements=None
  Three-Phase Series RLC Branch2 : spsThreePhaseSeriesRLCBranchLib/Three-Phase Series RLC Branch  LConnTagsString=A|B|C  RConnTagsString=A|B|C  BranchType=C  Resistance=rf(1)  Inductance=Lf(1)  Capacitance=Cf(3)  Measurements=None
  Three-Phase V-I Measurement : spsThreePhaseVIMeasurementLib/Three-Phase V-I Measurement  VoltageMeasurement=no  SetLabelV=off  LabelV=Vabc  Vpu=off  VpuLL=off  CurrentMeasurement=yes  SetLabelI=on  LabelI=Il3  Ipu=off  Pbase=100e6  Vbase=500e3  OutputType=Complex  PhasorSimulation=off  PSBequivalent=0
  Three-Phase V-I Measurement1 : spsThreePhaseVIMeasurementLib/Three-Phase V-I Measurement  VoltageMeasurement=phase-to-ground  SetLabelV=on  LabelV=Vo3  Vpu=off  VpuLL=off  CurrentMeasurement=yes  SetLabelI=on  LabelI=Io3  Ipu=off  Pbase=100e6  Vbase=500e3  OutputType=Complex  PhasorSimulation=off  PSBequivalent=0
  To Workspace : ToWorkspace  VariableName=xinv3  SampleTime=-1
      settings: MaxDataPoints=1  Save2DSignal=2-D array (concatenate along first dimension)
  Transfer Fcn : TransferFcn  Numerator=wc(3)  Denominator=[1 wc(3)]
  Transfer Fcn1 : TransferFcn  Numerator=wc(3)  Denominator=[1 wc(3)]
  Universal Bridge : spsUniversalBridgeLib/Universal Bridge  Arms=3  SnubberResistance=1e5  SnubberCapacitance=inf  Device=Average-model based VSC  Ron=1e-3  Lon=0  ForwardVoltages="[  0  0  ]"  ForwardVoltage=0  GTOparameters=[ 10e-6 , 20e-6 ]  IGBTparameters=[ 1e-6 , 2e-6 ]  Measurements=None  Measurements_2=None  converterType=Rectifier
  Voqref : Constant  Value=0
  abc to dq0 : spsabctodq0Lib/abc to dq0  Alignment=90 degrees behind phase A axis
  abc to dq1 : spsabctodq0Lib/abc to dq0  Alignment=90 degrees behind phase A axis
  abc to dq2 : spsabctodq0Lib/abc to dq0  Alignment=90 degrees behind phase A axis
  dq0 to abc : spsdq0toabcLib/dq0 to abc  Alignment=90 degrees behind phase A axis
  A : PMIOPort  Side=Right
  B : PMIOPort  Port=2  Side=Right
  C : PMIOPort  Port=3  Side=Right
  wires:
  [Vo3] -> abc to dq0/1
  abc to dq0/1 -> Demux/1
  Demux/1 -> [Vod]
  Demux/2 -> [Voq]
  Demux/3 -> Terminator/1
  Demux1/3 -> Terminator1/1
  Demux1/2 -> [Ioq]
  Demux1/1 -> [Iod]
  abc to dq1/1 -> Demux1/1
  [Io3] -> abc to dq1/1
  [Il3] -> abc to dq2/1
  Demux2/1 -> [Ild]
  abc to dq2/1 -> Demux2/1
  Demux2/2 -> [Ilq]
  Demux2/3 -> Terminator2/1
  [wt] -> abc to dq0/2, abc to dq1/2, abc to dq2/2
  [Voq] -> MATLAB Function/2(Voq)
  [Vod] -> MATLAB Function/1(Vod)
  [Iod] -> MATLAB Function/3(Iod)
  [Ioq] -> MATLAB Function/4(Ioq)
  MATLAB Function/1(p) -> Transfer Fcn/1
  MATLAB Function/2(q) -> Transfer Fcn1/1
  Constant/1 -> Sum/1
  Sum/1 -> Integrator/1
  Integrator/1 -> Sum9/2, [wt]
  [Vod] -> Sum2/3, Gain4/1
  Sum2/1 -> Subsystem2/1(e)
  Subsystem2/1(o) -> Sum3/2
  [Iod] -> Gain2/1
  Gain2/1 -> Sum3/1
  Voqref/1 -> Sum4/2
  [Voq] -> Gain5/1, Sum4/1
  Sum4/1 -> Subsystem3/1(e)
  Subsystem3/1(o) -> Sum5/2
  [Ioq] -> Gain3/1
  Gain3/1 -> Sum5/3
  Gain4/1 -> Sum5/1
  Gain5/1 -> Sum3/3
  Constant1/1 -> Sum2/2
  Gain8/1 -> Sum6/1
  Subsystem1/1(o) -> Sum6/2
  [Ilq] -> Sum8/1, Gain9/1
  [Ild] -> Sum7/2, Gain8/1
  Subsystem/1(o) -> Sum1/1
  Gain9/1 -> Sum1/2
  Sum3/1 -> Sum7/1
  Sum5/1 -> Sum8/2
  Sum7/1 -> Subsystem/1(e)
  Sum8/1 -> Subsystem1/1(e)
  Sum1/1 -> Mux/1
  Sum6/1 -> Mux/2
  Constant2/1 -> Mux/3
  Mux/1 -> Gain6/1
  Gain6/1 -> dq0 to abc/1
  [wt] -> dq0 to abc/2
  dq0 to abc/1 -> Delay/1, Demux3/1
  Demux3/1 -> Relational Operator/2
  Demux3/2 -> Relational Operator1/2
  Demux3/3 -> Relational Operator2/2
  Carrier/1 -> Relational Operator2/1, Relational Operator1/1, Relational Operator/1
  Relational Operator/1 -> Logical Operator/1, Mux1/1
  Relational Operator1/1 -> Logical Operator1/1, Mux1/3
  Relational Operator2/1 -> Logical Operator2/1, Mux1/5
  Logical Operator/1 -> Mux1/2
  Logical Operator1/1 -> Mux1/4
  Logical Operator2/1 -> Mux1/6
  Gain/1 -> Sum/2
  Transfer Fcn1/1 -> [Q], Scope1/2, Gain1/1
  Transfer Fcn/1 -> [P], Scope1/1, Gain/1
  Gain1/1 -> Sum2/1
  Sum9/1 -> [delta]
  [wt1] -> Sum9/1
  [xVoq] -> Mux2/5
  [xIlq] -> Mux2/7
  [Ioq] -> Mux2/13
  [Iod] -> Mux2/12
  [Voq] -> Mux2/11
  [Ild] -> Mux2/8
  [xIld] -> Mux2/6
  [Q] -> Mux2/3
  [P] -> Mux2/2
  [xVod] -> Mux2/4
  [Ilq] -> Mux2/9
  [delta] -> Mux2/1
  Mux2/1 -> To Workspace/1
  [Vod] -> Mux2/10
  Delay/1 -> Universal Bridge/1
  Subsystem1/2(x) -> [xIlq]
  Subsystem/2(x) -> [xIld]
  Subsystem2/2(x) -> [xVod]
  Subsystem3/2(x) -> [xVoq]
  connections:
  Three-Phase Series RLC Branch/LConn3 -- Universal Bridge/LConn3
  Three-Phase V-I Measurement/LConn3 -- Three-Phase Series RLC Branch/RConn3
  Three-Phase Series RLC Branch/RConn2 -- Three-Phase V-I Measurement/LConn2
  Three-Phase Series RLC Branch1/RConn3 -- C/RConn1
  Three-Phase Series RLC Branch/LConn2 -- Universal Bridge/LConn2
  Three-Phase Series RLC Branch2/LConn2 -- Three-Phase V-I Measurement1/LConn2 -- Three-Phase V-I Measurement/RConn2
  DC Voltage Source/RConn1 -- Universal Bridge/RConn1
  Three-Phase Series RLC Branch1/RConn2 -- B/RConn1
  Three-Phase Series RLC Branch2/LConn1 -- Three-Phase V-I Measurement1/LConn1 -- Three-Phase V-I Measurement/RConn1
  Three-Phase Series RLC Branch1/LConn1 -- Three-Phase V-I Measurement1/RConn1
  DC Voltage Source/LConn1 -- Universal Bridge/RConn2
  Three-Phase Series RLC Branch1/LConn2 -- Three-Phase V-I Measurement1/RConn2
  Three-Phase Series RLC Branch2/RConn2 -- Three-Phase Series RLC Branch2/RConn1 -- Three-Phase Series RLC Branch2/RConn3 -- Ground/LConn1
  Three-Phase Series RLC Branch2/LConn3 -- Three-Phase V-I Measurement1/LConn3 -- Three-Phase V-I Measurement/RConn3
  Universal Bridge/LConn1 -- Three-Phase Series RLC Branch/LConn1
  Three-Phase V-I Measurement/LConn1 -- Three-Phase Series RLC Branch/RConn1
  Three-Phase V-I Measurement1/RConn3 -- Three-Phase Series RLC Branch1/LConn3
  Three-Phase Series RLC Branch1/RConn1 -- A/RConn1

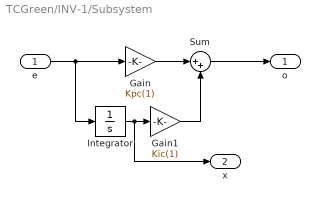
== system TCGreen/INV-1/Subsystem ==
  e : Inport
  Gain : Gain  Gain=Kpc(1)
  Gain1 : Gain  Gain=Kic(1)
  Integrator : Integrator
  Sum : Sum  Inputs=|++
  o : Outport
  x : Outport  Port=2
  wires:
  e/1 -> Integrator/1, Gain/1
  Gain/1 -> Sum/1
  Sum/1 -> o/1
  Integrator/1 -> x/1, Gain1/1
  Gain1/1 -> Sum/2

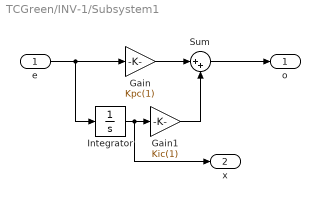
== system TCGreen/INV-1/Subsystem1 ==
  e : Inport
  Gain : Gain  Gain=Kpc(1)
  Gain1 : Gain  Gain=Kic(1)
  Integrator : Integrator
  Sum : Sum  Inputs=|++
  o : Outport
  x : Outport  Port=2
  wires:
  Gain1/1 -> Sum/2
  Integrator/1 -> Gain1/1, x/1
  Sum/1 -> o/1
  Gain/1 -> Sum/1
  e/1 -> Gain/1, Integrator/1

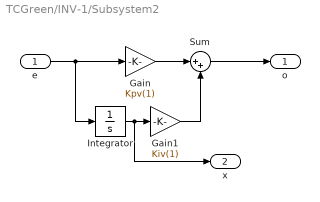
== system TCGreen/INV-1/Subsystem2 ==
  e : Inport
  Gain : Gain  Gain=Kpv(1)
  Gain1 : Gain  Gain=Kiv(1)
  Integrator : Integrator
  Sum : Sum  Inputs=|++
  o : Outport
  x : Outport  Port=2
  wires:
  Gain1/1 -> Sum/2
  Integrator/1 -> Gain1/1, x/1
  Sum/1 -> o/1
  Gain/1 -> Sum/1
  e/1 -> Gain/1, Integrator/1

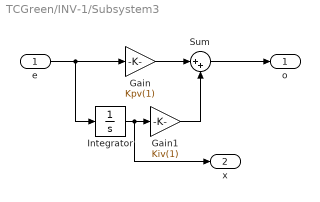
== system TCGreen/INV-1/Subsystem3 ==
  e : Inport
  Gain : Gain  Gain=Kpv(1)
  Gain1 : Gain  Gain=Kiv(1)
  Integrator : Integrator
  Sum : Sum  Inputs=|++
  o : Outport
  x : Outport  Port=2
  wires:
  e/1 -> Integrator/1, Gain/1
  Gain/1 -> Sum/1
  Sum/1 -> o/1
  Integrator/1 -> x/1, Gain1/1
  Gain1/1 -> Sum/2

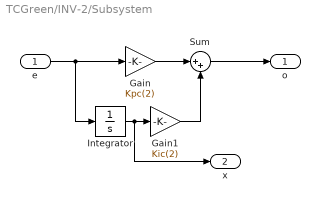
== system TCGreen/INV-2/Subsystem ==
  e : Inport
  Gain : Gain  Gain=Kpc(2)
  Gain1 : Gain  Gain=Kic(2)
  Integrator : Integrator
  Sum : Sum  Inputs=|++
  o : Outport
  x : Outport  Port=2
  wires:
  e/1 -> Integrator/1, Gain/1
  Gain/1 -> Sum/1
  Sum/1 -> o/1
  Integrator/1 -> x/1, Gain1/1
  Gain1/1 -> Sum/2

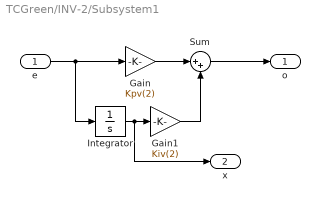
== system TCGreen/INV-2/Subsystem1 ==
  e : Inport
  Gain : Gain  Gain=Kpv(2)
  Gain1 : Gain  Gain=Kiv(2)
  Integrator : Integrator
  Sum : Sum  Inputs=|++
  o : Outport
  x : Outport  Port=2
  wires:
  e/1 -> Integrator/1, Gain/1
  Gain/1 -> Sum/1
  Sum/1 -> o/1
  Integrator/1 -> x/1, Gain1/1
  Gain1/1 -> Sum/2

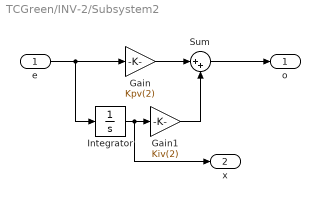
== system TCGreen/INV-2/Subsystem2 ==
  e : Inport
  Gain : Gain  Gain=Kpv(2)
  Gain1 : Gain  Gain=Kiv(2)
  Integrator : Integrator
  Sum : Sum  Inputs=|++
  o : Outport
  x : Outport  Port=2
  wires:
  Gain1/1 -> Sum/2
  Integrator/1 -> Gain1/1, x/1
  Sum/1 -> o/1
  Gain/1 -> Sum/1
  e/1 -> Gain/1, Integrator/1

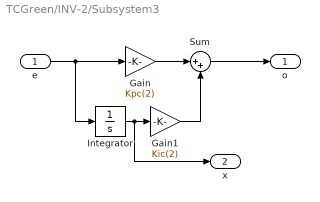
== system TCGreen/INV-2/Subsystem3 ==
  e : Inport
  Gain : Gain  Gain=Kpc(2)
  Gain1 : Gain  Gain=Kic(2)
  Integrator : Integrator
  Sum : Sum  Inputs=|++
  o : Outport
  x : Outport  Port=2
  wires:
  Gain1/1 -> Sum/2
  Integrator/1 -> Gain1/1, x/1
  Sum/1 -> o/1
  Gain/1 -> Sum/1
  e/1 -> Gain/1, Integrator/1

== system TCGreen/INV-3/Subsystem ==
  e : Inport
  Gain : Gain  Gain=Kpc(3)
  Gain1 : Gain  Gain=Kic(3)
  Integrator : Integrator
  Sum : Sum  Inputs=|++
  o : Outport
  x : Outport  Port=2
  wires:
  e/1 -> Integrator/1, Gain/1
  Gain/1 -> Sum/1
  Sum/1 -> o/1
  Integrator/1 -> x/1, Gain1/1
  Gain1/1 -> Sum/2

== system TCGreen/INV-3/Subsystem1 ==
  e : Inport
  Gain : Gain  Gain=Kpc(3)
  Gain1 : Gain  Gain=Kic(3)
  Integrator : Integrator
  Sum : Sum  Inputs=|++
  o : Outport
  x : Outport  Port=2
  wires:
  Gain1/1 -> Sum/2
  Integrator/1 -> Gain1/1, x/1
  Sum/1 -> o/1
  Gain/1 -> Sum/1
  e/1 -> Gain/1, Integrator/1

== system TCGreen/INV-3/Subsystem2 ==
  e : Inport
  Gain : Gain  Gain=Kpv(3)
  Gain1 : Gain  Gain=Kiv(3)
  Integrator : Integrator
  Sum : Sum  Inputs=|++
  o : Outport
  x : Outport  Port=2
  wires:
  Gain1/1 -> Sum/2
  Integrator/1 -> Gain1/1, x/1
  Sum/1 -> o/1
  Gain/1 -> Sum/1
  e/1 -> Gain/1, Integrator/1

== system TCGreen/INV-3/Subsystem3 ==
  e : Inport
  Gain : Gain  Gain=Kpv(3)
  Gain1 : Gain  Gain=Kiv(3)
  Integrator : Integrator
  Sum : Sum  Inputs=|++
  o : Outport
  x : Outport  Port=2
  wires:
  e/1 -> Integrator/1, Gain/1
  Gain/1 -> Sum/1
  Sum/1 -> o/1
  Integrator/1 -> x/1, Gain1/1
  Gain1/1 -> Sum/2

== matlab function TCGreen/INV-2/MATLAB Function ==
  data: Vod input; p output; Voq input; Iod input; Ioq input; q output
function [p,q] = fcn(Vod,Voq, Iod,Ioq)

p=1.5*(Vod*Iod+Voq*Ioq);
q=1.5*(Voq*Iod-Vod*Ioq);

== matlab function TCGreen/INV-1/MATLAB Function ==
  data: Vod input; p output; Voq input; Iod input; Ioq input; q output
function [p,q] = fcn(Vod,Voq, Iod,Ioq)

p=1.5*(Vod*Iod+Voq*Ioq);
q=1.5*(Voq*Iod-Vod*Ioq);

== matlab function TCGreen/INV-3/MATLAB Function ==
  data: Vod input; p output; Voq input; Iod input; Ioq input; q output
function [p,q] = fcn(Vod,Voq, Iod,Ioq)

p=1.5*(Vod*Iod+Voq*Ioq);
q=1.5*(Voq*Iod-Vod*Ioq);
